simulink model "plantModel"  (R2025b)
settings: Solver=VariableStepAuto  StartTime=0.0  StopTime=14  RelTol=1e-3
values from neighbouring files (symbols this model uses):
  a = 1.2    [vehicle_params.m]
  b = 1.6    [vehicle_params.m]
  beta_act = deg2rad(0.05)    [tests.m]    (also in vehicle_params.m = deg2rad(3))
  beta_th = deg2rad(1.0)    [tests.m]    (also in vehicle_params.m = deg2rad(6))
  Caf = 80000    [vehicle_params.m]
  Car = 80000    [vehicle_params.m]
  d = 0.75    [vehicle_params.m]
  Delta_a_y_gain = 0.4    [tests.m]    (also in vehicle_params.m = 0.1)
  Iz = 2500    [vehicle_params.m]
  k1 = 1.0    (= 1)    [tests.m]    (also in vehicle_params.m)
  k2 = 1.0    (= 1)    [tests.m]    (also in vehicle_params.m)
  Ki = 5000    [tests.m]    (also in vehicle_params.m)
  Kp = 3000    [tests.m]    (also in vehicle_params.m)
  L = a + b    (= 2.8)    [vehicle_params.m]
  m = 1500    [vehicle_params.m]
  Mz_max = 4000    [tests.m]    (also in vehicle_params.m)
  passive = 0    [tests.m]
  Rw = 0.30    (= 0.3)    [vehicle_params.m]
  use_sideslip_correction = 1    [tests.m]
  Vx = 20    [vehicle_params.m]
libraries: slpidlib x1
settings Model: Creator=jaiden  LastModifiedBy=jaiden

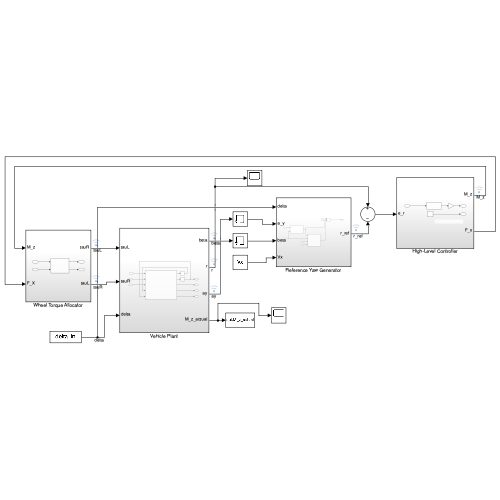
[thumbnail: Simulink's stored preview of the top-level diagram]
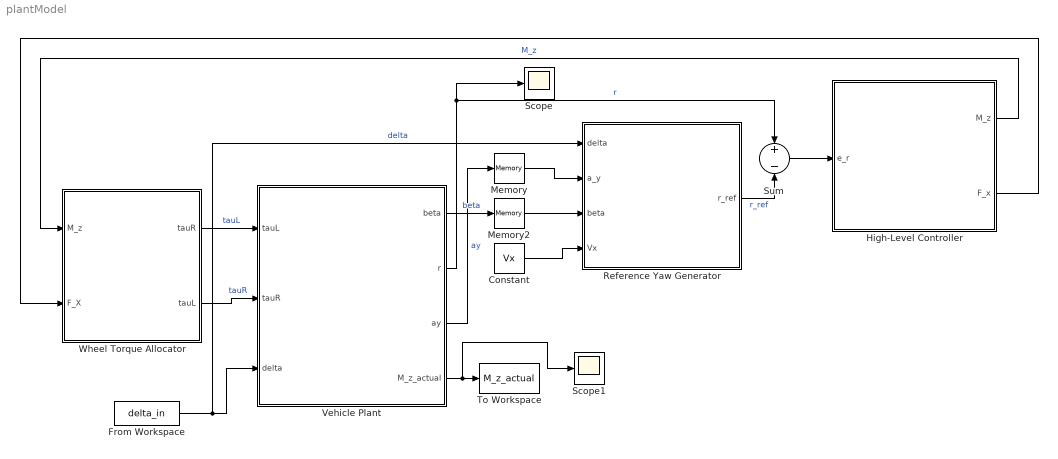
== system plantModel ==
  Constant : Constant  Value=Vx
  From Workspace : FromWorkspace  VariableName=delta_in
  High-Level Controller : Subsystem
  Memory : Memory
  Memory2 : Memory
  Reference Yaw Generator : Subsystem
  Scope : Scope
      settings: ActiveDisplayYMinimum=-1  ActiveDisplayYMaximum=1
  Scope1 : Scope
      settings: ActiveDisplayYMinimum=-2520.7331429053775  ActiveDisplayYMaximum=715.3256176936701
  Sum : Sum  Inputs=+-
  To Workspace : ToWorkspace  VariableName=M_z_actual  SaveFormat=Timeseries  SampleTime=-1
  Vehicle Plant : Subsystem
  Wheel Torque Allocator : Subsystem
  wires:
  High-Level Controller/1(M_z) -> Wheel Torque Allocator/1(M_z)  "M_z"
  Sum/1 -> High-Level Controller/1(e_r)
  Reference Yaw Generator/1(r_ref) -> Sum/2  "r_ref"
  Constant/1 -> Reference Yaw Generator/4(Vx)
  Memory2/1 -> Reference Yaw Generator/3(beta)
  Wheel Torque Allocator/2(tauL) -> Vehicle Plant/2(tauR)  "tauR"
  Memory/1 -> Reference Yaw Generator/2(a_y)
  Vehicle Plant/3(ay) -> Memory/1  "ay"
  High-Level Controller/2(F_x) -> Wheel Torque Allocator/2(F_X)
  Vehicle Plant/2(r) -> Scope/1, Sum/1  "r"
  Vehicle Plant/1(beta) -> Memory2/1  "beta"
  From Workspace/1 -> Vehicle Plant/3(delta), Reference Yaw Generator/1(delta)  "delta"
  Vehicle Plant/4(M_z_actual) -> Scope1/1, To Workspace/1
  Wheel Torque Allocator/1(tauR) -> Vehicle Plant/1(tauL)  "tauL"

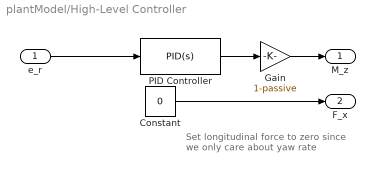
== system plantModel/High-Level Controller ==
  note: Set longitudinal force to zero since
      | we only care about yaw rate
  e_r : Inport
  Constant : Constant  Value=0
  Gain : Gain  Gain=1-passive
  PID Controller : slpidlib/PID Controller  Controller=PID  Form=Parallel  TimeDomain=Continuous-time  UseExternalTs=off  SampleTime=-1  IntegratorMethod=Forward Euler  FilterMethod=Forward Euler  ControllerParametersSource=internal  P=Kp  I=Ki  UseKiTs=off  D=0  UseExternalDerivativeSource=off  N=100  UseFilter=on  TunerSelectOption=Transfer Function Based (PID Tuner App)  InitialConditionSource=internal  InitialConditionForIntegrator=0  InitialConditionForFilter=0  DifferentiatorICPrevScaledInput=0  ExternalReset=none  TrackingMode=off  Kt=1  LimitOutput=on  SatLimitsSource=internal  UpperSaturationLimit=Mz_max  LowerSaturationLimit=-Mz_max  LinearizeAsGain=on  AntiWindupMode=none  Kb=1  LimitIntegrator=off  UpperIntegratorSaturationLimit=inf  LowerIntegratorSaturationLimit=-inf  POutMin=[]  POutMax=[]  IOutMin=[]  IOutMax=[]  DOutMin=[]  DOutMax=[]  NOutMin=[]  NOutMax=[]  SumOutMin=[]  SumOutMax=[]  SaturationOutMin=[]  SaturationOutMax=[]  PParamMin=[]  PParamMax=[]  IParamMin=[]  IParamMax=[]  DParamMin=[]  DParamMax=[]  NParamMin=[]  NParamMax=[]  KbParamMin=[]  KbParamMax=[]  KtParamMin=[]  KtParamMax=[]  KbOutMin=[]  KbOutMax=[]  KtOutMin=[]  KtOutMax=[]  IntegratorOutMin=[]  IntegratorOutMax=[]  FilterOutMin=[]  FilterOutMax=[]  SumI1OutMin=[]  SumI1OutMax=[]  SumI2OutMin=[]  SumI2OutMax=[]  SumI3OutMin=[]  SumI3OutMax=[]  SumI4OutMin=[]  SumI4OutMax=[]  SumDOutMin=[]  SumDOutMax=[]  DifferentiatorOutMin=[]  DifferentiatorOutMax=[]  FilterDiffOutCoefMin=[]  FilterDiffOutCoefMax=[]  ReciprocalOutMin=[]  ReciprocalOutMax=[]  SumDenOutMin=[]  SumDenOutMax=[]  SumNumOutMin=[]  SumNumOutMax=[]  DivideOutMin=[]  DivideOutMax=[]  UdiffTsProdOutMin=[]  UdiffTsProdOutMax=[]  NTsProdOutMin=[]  NTsProdOutMax=[]  UintegralTsProdOutMin=[]  UintegralTsProdOutMax=[]  UngainTsProdOutMin=[]  UngainTsProdOutMax=[]  ClampingZeroOutDataTypeStr=Inherit: Inherit via back propagation  ClampingZeroOutMin=[]  ClampingZeroOutMax=[]  FilterDenConstantOutDataTypeStr=Inherit: Inherit via back propagation  FilterDenConstantOutMin=[]  FilterDenConstantOutMax=[]  PCopyOutDataTypeStr=Inherit: Inherit via back propagation  PCopyOutMin=[]  PCopyOutMax=[]  NCopyOutDataTypeStr=Inherit: Inherit via back propagation  NCopyOutMin=[]  NCopyOutMax=[]  IntegratorContinuousStateAttributes=''  IntegratorStateMustResolveToSignalObject=off  IntegratorRTWStateStorageClass=Auto  FilterContinuousStateAttributes=''  FilterStateMustResolveToSignalObject=off  FilterRTWStateStorageClass=Auto  ParallelPVariant=InternalParameters  IdealPVariant=Disabled  IVariant=InternalParameters  DVariant=InternalParameters  IntegratorVariant=Continuous  SatVariant=Enabled  AWVariant=Passthrough  PCopyVariant=Disabled  TRVariant=Disabled  FdbkBlocksVariant=Forward  IdealPFdbkVariant=Disabled  SatFdbkVariant=Disabled  DerivativeFilterVariant=ContFilter  NVariant=InternalParameters  NCopyVariant=Disabled  FilterICVariant=InternalICsFilter  IntegratorICVariant=InternalICs  ExternalResetVariant=Disabled  TRSumVariant=Passthrough  SumFdbkVariant=Disabled  SumVariant=Sum_PID  TsampFilterVariant=InternalTs  TsampNgainVariant=Passthrough  TsampIntegralVariant=Disabled_SignalSpec  ExternalSaturationOutDataTypeStr=Inherit: Same as second input  DerivativeSourceVariant=ErrorSignal  PreIntVariant=InternalPreInt
  M_z : Outport
  F_x : Outport  Port=2
  wires:
  e_r/1 -> PID Controller/1
  Constant/1 -> F_x/1
  PID Controller/1 -> Gain/1
  Gain/1 -> M_z/1

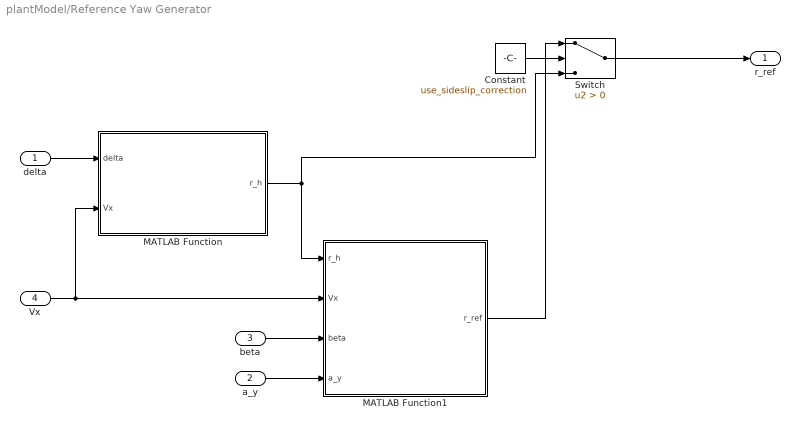
== system plantModel/Reference Yaw Generator ==
  delta : Inport
  a_y : Inport  Port=2
  beta : Inport  Port=3
  Vx : Inport  Port=4
  Constant : Constant  Value=use_sideslip_correction
  MATLAB Function : MATLAB Function  TreatAsAtomicUnit=on
  MATLAB Function1 : MATLAB Function  TreatAsAtomicUnit=on
  Switch : Switch  Criteria=u2 > Threshold  SaturateOnIntegerOverflow=off  InputSameDT=off
  r_ref : Outport
  wires:
  MATLAB Function1/1(r_ref) -> Switch/1
  a_y/1 -> MATLAB Function1/4(a_y)
  Vx/1 -> MATLAB Function/2(Vx), MATLAB Function1/2(Vx)
  beta/1 -> MATLAB Function1/3(beta)
  MATLAB Function/1(r_h) -> Switch/3, MATLAB Function1/1(r_h)
  delta/1 -> MATLAB Function/1(delta)
  Constant/1 -> Switch/2
  Switch/1 -> r_ref/1

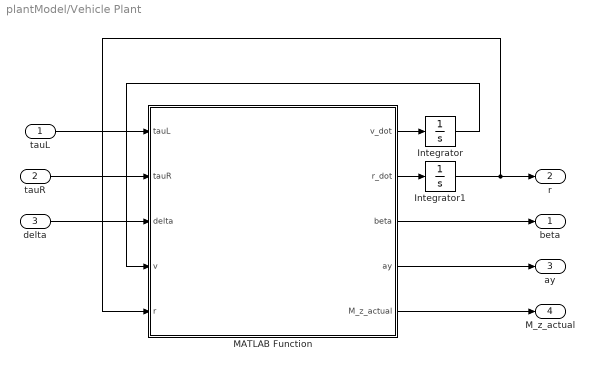
== system plantModel/Vehicle Plant ==
  tauL : Inport
  tauR : Inport  Port=2
  delta : Inport  Port=3
  Integrator : Integrator
  Integrator1 : Integrator
  MATLAB Function : MATLAB Function  TreatAsAtomicUnit=on
  beta : Outport
  r : Outport  Port=2
  ay : Outport  Port=3
  M_z_actual : Outport  Port=4
  wires:
  tauL/1 -> MATLAB Function/1(tauL)
  delta/1 -> MATLAB Function/3(delta)
  tauR/1 -> MATLAB Function/2(tauR)
  MATLAB Function/1(v_dot) -> Integrator/1
  Integrator/1 -> MATLAB Function/4(v)
  MATLAB Function/2(r_dot) -> Integrator1/1
  Integrator1/1 -> MATLAB Function/5(r), r/1
  MATLAB Function/3(beta) -> beta/1
  MATLAB Function/4(ay) -> ay/1
  MATLAB Function/5(M_z_actual) -> M_z_actual/1

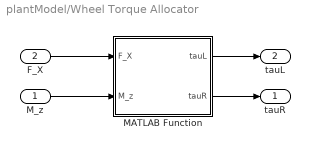
== system plantModel/Wheel Torque Allocator ==
  M_z : Inport
  F_X : Inport  Port=2
  MATLAB Function : MATLAB Function  TreatAsAtomicUnit=on
  tauR : Outport
  tauL : Outport  Port=2
  wires:
  M_z/1 -> MATLAB Function/2(M_z)
  F_X/1 -> MATLAB Function/1(F_X)
  MATLAB Function/2(tauR) -> tauR/1
  MATLAB Function/1(tauL) -> tauL/1

== matlab function plantModel/Wheel Torque Allocator/MATLAB Function ==
  data: F_X input; tauL output; M_z input; tauR output; d parameter; Rw parameter
function [tauL, tauR] = torque_allocator(F_X, M_z, d, Rw)

tauL = 0.5*(F_X - M_z/d)*Rw;
tauR = 0.5*(F_X + M_z/d)*Rw;

end

== matlab function plantModel/Vehicle Plant/MATLAB Function ==
  data: tauL input; v_dot output; tauR input; delta input; r_dot output; beta output; ay output; M_z_actual output; v input; r input; m parameter; Iz parameter; a parameter; b parameter; d parameter; Rw parameter; Caf parameter; Car parameter; Vx parameter
function [v_dot,r_dot, beta, ay, M_z_actual] = vehicle_dynamics(tauL, tauR, delta, v, r, m, Iz, a, b, d, Rw, Caf, Car, Vx)
% vehicle_dynamics
% Single-track linear handling model (from lecture 4 slides) w/ direct yaw
% moment input.
%
% Inputs:
%   tauL    = left-side wheel torque [N*m]
%   tauR    = right-side wheel torque [N*m]
%   delta   = steering angle [rad]
%   v       = lateral velocity [m/s]
%   r = yaw rate [rad/s]
%
% Outputs:
%   v_dot       = lateral acceleration [m/s^2]
%   r_dot       = yaw acceleration [rad/s^2]
%   beta        = sideslip angle [rad]
%   ay          = lateral acceleration [m/s^2]
%   M_z_actual  = yaw moment from torque vectoring[N*m]

% Calculate yaw moment from torque difference
M_z_actual = (d/Rw)*(tauR - tauL);

% Tire slip angles
alpha_f = delta - (v + a*r)/Vx;
alpha_r = -(v - b*r)/Vx;

% Linear tire forces
Fyf = Caf * alpha_f;
Fyr = Car * alpha_r;

% Lateral dynamics
v_dot = (Fyf + Fyr)/m - Vx*r;

% Yaw dynamics
r_dot = (a*Fyf - b*Fyr + M_z_actual)/Iz;

% Sideslip angle
beta = -atan(v/Vx);

% Lateral acceleration
ay = v_dot + Vx*r;

end

== matlab function plantModel/Reference Yaw Generator/MATLAB Function ==
  data: delta input; r_h output; Vx input; m parameter; L parameter; a parameter; b parameter; Caf parameter; Car parameter
function r_h = handling_yaw_rate(delta, Vx, m, L, a, b, Caf, Car)

% page 49 lecture 4 slides
kus = m/(L*Caf*Car)*(b*Car - a*Caf);
% page 52 lecture 4 slides
r_h = (Vx/(L + kus*Vx^2))*delta;

end

== matlab function plantModel/Reference Yaw Generator/MATLAB Function1 ==
  data: r_h input; Vx input; r_ref output; beta input; beta_act parameter; beta_th parameter; k1 parameter; k2 parameter; Delta_a_y_gain parameter; a_y input
function r_ref = sideslip_correction(r_h, Vx, beta, beta_act, beta_th, k1, k2, Delta_a_y_gain, a_y)

Delta_a_y = Delta_a_y_gain * abs(a_y);

r_sat = (a_y - sign(a_y)*Delta_a_y)/Vx; % paper eq (5)

% paper eq (4)
if abs(r_h) < abs(r_sat)
    r_s = r_h;
else
    r_s = abs(r_sat) * sign(r_h);
end

% paper eq (3)
if abs(beta) < beta_act
    F = 0;
elseif abs(beta) <= beta_th
    F = k1*(abs(beta) - beta_act)/(beta_th - beta_act);
else
    F = k2;
end

r_ref = r_h - F*(r_h - r_s);

end
